simulink model "BLDCmotorControl_FOC_R2017b_fixdt"  (R2017b)
settings: Solver=FixedStepDiscrete  StartTime=0  StopTime=0.5  FixedStep=Ts  MaxStep=1e-6  RelTol=1e-6  AbsTol=1e-6  EnableMultiTasking=on
PreLoadFcn:
  | addpath(pwd);
  | addpath(genpath('01_Libraries'));
  | addpath(genpath('02_Figures'));
  | addpath(genpath('03_CreateParamTable'));
InitFcn:
  | init_model;
values from neighbouring files (symbols this model uses):
  a_elecAngle = 60    [init_model.m]
  a_elecPeriod = 360    [init_model.m]
  a_phaAdvMax = 25    [init_model.m]
  b_diagEna = 1    [init_model.m]
  b_fieldWeakEna = 0    [init_model.m]
  cf_currFilt = 0.12    [init_model.m]
  cf_idKi = 60 / (f_ctrl/3)    (= 0.01125)    [init_model.m]
  cf_idKp = 0.2    [init_model.m]
  cf_iqKi = 100 / (f_ctrl/3)    (= 0.01875)    [init_model.m]
  cf_iqKiLimProt = 60 / (f_ctrl/3)    (= 0.01125)    [init_model.m]
  cf_iqKp = 0.3    [init_model.m]
  cf_KbLimProt = 1000 / (f_ctrl/3)    (= 0.1875)    [init_model.m]
  cf_nKi = 20.4 / (f_ctrl/3)    (= 0.003825)    [init_model.m]
  cf_nKiLimProt = 20 / (f_ctrl/3)    (= 0.00375)    [init_model.m]
  cf_nKp = 1.18    [init_model.m]
  cf_speedCoef = round(f_ctrl * a_mechAngle * (pi/180) * (30/pi))    [init_model.m]
  CTRL_COM = 0    [init_model.m]
  CTRL_FOC = 2    [init_model.m]
  CTRL_SIN = 1    [init_model.m]
  dV_openRate = 1000 / (f_ctrl/3)    (= 0.1875)    [init_model.m]
  dz_cntTrnsDetHi = 40    [init_model.m]
  dz_cntTrnsDetLo = 20    [init_model.m]
  i_max = i_max * i_sca    (= 750)    [init_model.m]
  id_fieldWeakMax = 5 * i_sca    (= 250)    [init_model.m]
  iq_maxSca_M1 = sqrt(1 - iq_maxSca_XA.^2)    [init_model.m]
  n_commAcvLo = 15    [init_model.m]
  n_commDeacvHi = 30    [init_model.m]
  n_fieldWeakAuthHi = 400    [init_model.m]
  n_fieldWeakAuthLo = 300    [init_model.m]
  n_max = 1000    [init_model.m]
  n_polePairs = 15    [init_model.m]
  n_stdStillDet = 3    [init_model.m]
  OPEN_MODE = 0    [init_model.m]
  r_cos_M1 = cos((a_elecAngle_XA + 0)*(pi/180))    [init_model.m]
  r_errInpTgtThres = 600    [init_model.m]
  r_fieldWeakHi = 1500    [init_model.m]
  r_fieldWeakLo = 1000    [init_model.m]
  r_sin3PhaA_M1 = sin3Arm + A*r_sinPhaA_M1    [init_model.m]
  r_sin3PhaB_M1 = sin3Arm + A*r_sinPhaB_M1    [init_model.m]
  r_sin3PhaC_M1 = sin3Arm + A*r_sinPhaC_M1    [init_model.m]
  r_sin_M1 = sin((a_elecAngle_XA + 0)*(pi/180))    [init_model.m]
  SPD_MODE = 2    [init_model.m]
  t_errDequal = 1.80 * f_ctrl/3    (= 9600)    [init_model.m]
  t_errQual = 0.24 * f_ctrl/3    (= 1280)    [init_model.m]
  TRQ_MODE = 3    [init_model.m]
  Ts = 5e-6    (= 5e-06)    [init_model.m]
  Ts_ctrl = 6e-5    (= 6e-05)    [init_model.m]
  Vd_max = 1000 - V_margin    (= 900)    [init_model.m]
  vec_hallToPos = [0 2 0 1 4 3 5 0]    [init_model.m]
  VLT_MODE = 1    [init_model.m]
  Vq_max_M1 = sqrt(Vd_max^2 - Vq_max_XA.^2)    [init_model.m]
  z_commutMap_M1 = [-1 -1  0  1  1  0 ... (first row only)    [init_model.m]
  z_ctrlModReq = VLT_MODE    (= 1)    [init_model.m]
  z_ctrlTypSel = 2    [init_model.m]
  z_maxCntRst = 2000    [init_model.m]
  z_selPhaCurMeasABC = 0    [init_model.m]
undefined symbols (not defined in the file or in its folder): DiscIntNeverNeededParam, sigbuilder_block
libraries: BLDC_controller_Lib x15, simulink x14, powerlib x6, pePwmGenerator x1
(part 4 of 4)

== system BLDCmotorControl_FOC_R2017b_fixdt/BLDC_controller/F05_Field_Oriented_Control/Clarke_Transform/Clarke_PhasesBC ==
  note: Clarke Transform:
      | i_alpha = - i_phaB - i_phaC
      | i_beta = (1/sqrt(3)) * (i_phaB - i_phaC)
  i_phaB : Inport
  i_phaC : Inport  Port=2
  Action Port : ActionPort  ActionType=elseif
  Gain2 : Gain  Tag=struct('comment',struct('text','','placement',1),'logdata',struct('maxnumvals',inf,'plotchannels',[],'loggingmode',3,'channels',1),'output',struct('variable','','description','','name','$S_$B','width',1,'address','','max',NaN,'min',NaN,'class','default','type','CONTINUOUS','scaling','','lsb',1,'offset',0,'arb',0,'freeze',1,'unit','','autoscalingmode',1,'lowerheadroom',1,'upperheadroom',1,'headroomunit','bit','keepdatatype',1,'checkmin',0,'checkmax',0,'castoutput',0,'show',0),'gain',struct('variable','','description','','name','$S_$B_gain','width',1,'address','','max',NaN,'min',NaN,'class','default','type','CONTINUOUS','scaling','','lsb',1,'offset',0,'arb',0,'freeze',1,'unit','','keepdatatype',1,'value','1','scalar',0,'tolerance',1),'scalingvalid',0,'date',730486)  Gain=1/sqrt(3)  RndMeth=Zero  OutDataTypeStr=Inherit: Same as input
  Sum1 : Sum  Inputs=--  OutDataTypeStr=fixdt(1,16,4)  RndMeth=Simplest  SaturateOnIntegerOverflow=on
  Sum3 : Sum  Inputs=+-  OutDataTypeStr=fixdt(1,16,4)  RndMeth=Simplest  SaturateOnIntegerOverflow=on
  i_alphaBC : Outport
  i_betaBC : Outport  Port=2
  wires:
  [i_phaC] -> Sum1/2
  [i_phaB] -> Sum1/1
  [i_phaC] -> Sum3/2
  Gain2/1 -> i_betaBC/1
  Sum3/1 -> Gain2/1
  [i_phaB] -> Sum3/1
  Sum1/1 -> i_alphaBC/1
  i_phaB/1 -> [i_phaB]
  i_phaC/1 -> [i_phaC]

== system BLDCmotorControl_FOC_R2017b_fixdt/BLDC_controller/F05_Field_Oriented_Control/FOC/Open_Mode ==
  note: Just copy the target which will be reduced to 0 in the Input_Target_Sythesis function.
  r_inpTgtSca : Inport
  Action Port : ActionPort  ActionType=default
  Vq_Open : Outport
  wires:
  r_inpTgtSca/1 -> Vq_Open/1

== system BLDCmotorControl_FOC_R2017b_fixdt/BLDC_controller/F05_Field_Oriented_Control/FOC/Speed_Mode ==
  note: The input is scaled, so already between [n_min, n_max]
  r_inpTgtSca : Inport
  Vq_max : Inport  Port=2
  Vq_min : Inport  Port=3
  n_mot : Inport  Port=4
  iq_limProtErr : Inport  Port=5
  Action Port : ActionPort  ActionType=case
  PI_clamp_fixdt : BLDC_controller_Lib/PI_clamp_fixdt  SystemSampleTime=-1
  Sum3 : Sum  Inputs=|+-  RndMeth=Simplest  SaturateOnIntegerOverflow=on
  cf_nKi : Constant  Value=cf_nKi  VectorParams1D=off  OutDataTypeStr=fixdt(0,16,16)
  cf_nKp : Constant  Value=cf_nKp  OutDataTypeStr=fixdt(0,16,12)
  Vq_Spd : Outport
  wires:
  cf_nKi/1 -> PI_clamp_fixdt/3
  cf_nKp/1 -> PI_clamp_fixdt/2
  [n_mot] -> Sum3/2
  Sum3/1 -> PI_clamp_fixdt/1
  r_inpTgtSca/1 -> [r_inpTgtSca]
  Vq_max/1 -> [Vq_max]
  Vq_min/1 -> [Vq_min]
  n_mot/1 -> [n_mot]
  [r_inpTgtSca] -> Sum3/1
  iq_limProtErr/1 -> [iq_limProtErr]
  [iq_limProtErr] -> PI_clamp_fixdt/6
  PI_clamp_fixdt/1 -> Vq_Spd/1
  [Vq_min] -> PI_clamp_fixdt/5
  [Vq_max] -> PI_clamp_fixdt/4

== system BLDCmotorControl_FOC_R2017b_fixdt/BLDC_controller/F05_Field_Oriented_Control/FOC/Torque_Mode ==
  r_inpTgtSca : Inport
  Vq_max : Inport  Port=2
  Vq_min : Inport  Port=3
  iq : Inport  Port=4
  iq_max : Inport  Port=5
  iq_min : Inport  Port=6
  Vq_nLimProtMax : Inport  Port=7
  Action Port : ActionPort  ActionType=case
  Gain4 : Gain  Tag=struct('comment',struct('text','','placement',1),'logdata',struct('maxnumvals',inf,'plotchannels',[],'loggingmode',3,'channels',1),'output',struct('variable','','description','','name','$S_$B','width',1,'address','','max',NaN,'min',NaN,'class','default','type','CONTINUOUS','scaling','','lsb',1,'offset',0,'arb',0,'freeze',1,'unit','','autoscalingmode',1,'lowerheadroom',1,'upperheadroom',1,'headroomunit','bit','keepdatatype',1,'checkmin',0,'checkmax',0,'castoutput',0,'show',0),'gain',struct('variable','','description','','name','$S_$B_gain','width',1,'address','','max',NaN,'min',NaN,'class','default','type','CONTINUOUS','scaling','','lsb',1,'offset',0,'arb',0,'freeze',1,'unit','','keepdatatype',1,'value','1','scalar',0,'tolerance',1),'scalingvalid',0,'date',730486)  Gain=-1  RndMeth=Zero  OutDataTypeStr=Inherit: Same as input  ParamDataTypeStr=Inherit: Same as input
  MinMax1 : MinMax  Inputs=2
  MinMax2 : MinMax  Function=max  Inputs=2
  PI_clamp_fixdt : BLDC_controller_Lib/PI_clamp_fixdt  SystemSampleTime=-1
  Saturation Dynamic1 : simulink/Discontinuities/Saturation Dynamic  OutMin=[]  OutMax=[]  OutDataTypeStr=Inherit: Same as second input  OutDataType=fixdt(1, 16)  OutScaling=2^-10  DoSatur=off
  Sum2 : Sum  Inputs=|+-  RndMeth=Simplest  SaturateOnIntegerOverflow=on
  cf_iqKi : Constant  Value=cf_iqKi  OutDataTypeStr=fixdt(0,16,16)
  cf_iqKp : Constant  Value=cf_iqKp  OutDataTypeStr=fixdt(0,16,12)
  constant2 : Constant  Value=0  OutDataTypeStr=Inherit: Inherit via back propagation
  Vq_Trq : Outport
  wires:
  Vq_max/1 -> [Vq_max]
  r_inpTgtSca/1 -> [r_inpTgtSca]
  Vq_min/1 -> [Vq_min]
  iq/1 -> [iq]
  iq_min/1 -> [iq_min]
  iq_max/1 -> [iq_max]
  Vq_nLimProtMax/1 -> [Vq_nLimProtMax]
  [r_inpTgtSca] -> Saturation Dynamic1/2
  constant2/1 -> PI_clamp_fixdt/6
  Saturation Dynamic1/1 -> Sum2/1
  PI_clamp_fixdt/1 -> Vq_Trq/1
  [iq_max] -> Saturation Dynamic1/1
  [iq_min] -> Saturation Dynamic1/3
  cf_iqKp/1 -> PI_clamp_fixdt/2
  Sum2/1 -> PI_clamp_fixdt/1
  [iq] -> Sum2/2
  [Vq_minTrq] -> PI_clamp_fixdt/5
  [Vq_maxTrq] -> PI_clamp_fixdt/4
  cf_iqKi/1 -> PI_clamp_fixdt/3
  [Vq_nLimProtMax] -> MinMax1/2, Gain4/1
  [Vq_max] -> MinMax1/1
  Gain4/1 -> MinMax2/1
  [Vq_min] -> MinMax2/2
  MinMax1/1 -> [Vq_maxTrq]
  MinMax2/1 -> [Vq_minTrq]

== system BLDCmotorControl_FOC_R2017b_fixdt/BLDC_controller/F05_Field_Oriented_Control/FOC/Vd_Calculation ==
  id_Tgt : Inport
  id : Inport  Port=2
  Vd_max : Inport  Port=3
  Vd_min : Inport  Port=4
  id_max : Inport  Port=5
  id_min : Inport  Port=6
  Action Port : ActionPort  ActionType=then
  PI_clamp_fixdt : BLDC_controller_Lib/PI_clamp_fixdt  SystemSampleTime=-1
  Saturation Dynamic : simulink/Discontinuities/Saturation Dynamic  OutMin=[]  OutMax=[]  OutDataTypeStr=Inherit: Same as second input  OutDataType=fixdt(1, 16)  OutScaling=2^-10  DoSatur=off
  Sum3 : Sum  Inputs=|+-  RndMeth=Simplest  SaturateOnIntegerOverflow=on
  cf_idKi1 : Constant  Value=cf_idKi  OutDataTypeStr=fixdt(0,16,16)
  cf_idKp1 : Constant  Value=cf_idKp  OutDataTypeStr=fixdt(0,16,12)
  constant1 : Constant  Value=0  OutDataTypeStr=Inherit: Inherit via back propagation
  Vd : Outport
  wires:
  [id] -> Sum3/2
  [id_Tgt] -> Saturation Dynamic/2
  id_Tgt/1 -> [id_Tgt]
  id/1 -> [id]
  Vd_min/1 -> [Vd_min]
  Vd_max/1 -> [Vd_max]
  id_max/1 -> [id_max]
  id_min/1 -> [id_min]
  Saturation Dynamic/1 -> Sum3/1
  [id_max] -> Saturation Dynamic/1
  [id_min] -> Saturation Dynamic/3
  Sum3/1 -> PI_clamp_fixdt/1
  PI_clamp_fixdt/1 -> Vd/1
  cf_idKp1/1 -> PI_clamp_fixdt/2
  cf_idKi1/1 -> PI_clamp_fixdt/3
  constant1/1 -> PI_clamp_fixdt/6
  [Vd_min] -> PI_clamp_fixdt/5
  [Vd_max] -> PI_clamp_fixdt/4

== system BLDCmotorControl_FOC_R2017b_fixdt/BLDC_controller/F05_Field_Oriented_Control/FOC/Voltage_Mode ==
  r_inpTgtSca : Inport
  r_inpTgtScaAbs : Inport  Port=2
  Vq_max : Inport  Port=3
  Vq_min : Inport  Port=4
  r_iqLimProtMax : Inport  Port=5
  r_nLimProtMax : Inport  Port=6
  Action Port : ActionPort  ActionType=case
  Divide1 : Product  Inputs=**  RndMeth=Simplest  OutDataTypeStr=Inherit: Same as first input
  MinMax : MinMax  Inputs=3
  Saturation Dynamic1 : simulink/Discontinuities/Saturation Dynamic  OutMin=[]  OutMax=[]  OutDataTypeStr=Inherit: Same as second input  OutDataType=fixdt(1, 16)  OutScaling=2^-10  DoSatur=off
  SignDeltaU2 : Signum  DisableCoverage=on
  Signal Conversion2 : SignalConversion  OverrideOpt=off
  Vq_Vlt : Outport
  wires:
  r_inpTgtSca/1 -> [r_inpTgtSca]
  [Vq_min] -> Saturation Dynamic1/3
  [Vq_max] -> Saturation Dynamic1/1
  Vq_max/1 -> [Vq_max]
  Vq_min/1 -> [Vq_min]
  r_iqLimProtMax/1 -> [r_iqLimProtMax]
  r_nLimProtMax/1 -> [r_nLimProtMax]
  Signal Conversion2/1 -> Vq_Vlt/1
  Saturation Dynamic1/1 -> Signal Conversion2/1
  [r_nLimProtMax] -> MinMax/3
  [r_iqLimProtMax] -> MinMax/2
  r_inpTgtScaAbs/1 -> [r_inpTgtScaAbs]
  [r_inpTgtScaAbs] -> MinMax/1
  [r_inpTgtSca] -> SignDeltaU2/1
  MinMax/1 -> Divide1/1
  SignDeltaU2/1 -> Divide1/2
  Divide1/1 -> Saturation Dynamic1/2

== system BLDCmotorControl_FOC_R2017b_fixdt/BLDC_controller/F05_Field_Oriented_Control/Motor_Limitations/Speed_Mode_Protection ==
  iq : Inport
  iq_max : Inport  Port=2
  iq_min : Inport  Port=3
  Action Port : ActionPort  ActionType=case
  Divide1 : Product  Inputs=**  OutDataTypeStr=fixdt(1,32,20)  RndMeth=Simplest
  Saturation Dynamic : simulink/Discontinuities/Saturation Dynamic  OutMin=[]  OutMax=[]  OutDataTypeStr=Inherit: Same as second input  OutDataType=fixdt(1, 16)  OutScaling=2^-10  DoSatur=off
  Sum3 : Sum  Inputs=|+-  RndMeth=Simplest
  cf_iqKiLimProt : Constant  Value=cf_iqKiLimProt  OutDataTypeStr=fixdt(0,16,16)
  iq_limProtErr : Outport  InitialOutput=0
  wires:
  iq/1 -> Sum3/2, Saturation Dynamic/2
  Saturation Dynamic/1 -> Sum3/1
  iq_max/1 -> Saturation Dynamic/1
  iq_min/1 -> Saturation Dynamic/3
  cf_iqKiLimProt/1 -> Divide1/2
  Divide1/1 -> iq_limProtErr/1
  Sum3/1 -> Divide1/1

== system BLDCmotorControl_FOC_R2017b_fixdt/BLDC_controller/F05_Field_Oriented_Control/Motor_Limitations/Torque_Mode_Protection ==
  n_motAbs : Inport
  n_max : Inport  Port=2
  Vq_max : Inport  Port=3
  Action Port : ActionPort  ActionType=case
  Constant1 : Constant  Value=0  OutDataTypeStr=Inherit: Inherit via back propagation
  I_backCalc_fixdt : BLDC_controller_Lib/I_backCalc_fixdt  yInit=0
      settings: AttributesFormatString=Ini=%<yInit>
  Sum1 : Sum  Inputs=+-  RndMeth=Simplest  OutDataTypeStr=Inherit: Same as first input
  cf_KbLimProt : Constant  Value=cf_KbLimProt  OutDataTypeStr=fixdt(0,16,12)
  cf_nKiLimProt : Constant  Value=cf_nKiLimProt  OutDataTypeStr=fixdt(0,16,16)
  Vq_nLimProtMax : Outport  InitialOutput=0
  wires:
  n_motAbs/1 -> [n_motAbs]
  n_max/1 -> [n_max]
  Sum1/1 -> I_backCalc_fixdt/1
  [n_motAbs] -> Sum1/2
  Constant1/1 -> I_backCalc_fixdt/5
  [n_max] -> Sum1/1
  cf_nKiLimProt/1 -> I_backCalc_fixdt/2
  cf_KbLimProt/1 -> I_backCalc_fixdt/3
  [Vq_max] -> I_backCalc_fixdt/4
  I_backCalc_fixdt/1 -> Vq_nLimProtMax/1
  Vq_max/1 -> [Vq_max]

== system BLDCmotorControl_FOC_R2017b_fixdt/BLDC_controller/F05_Field_Oriented_Control/Motor_Limitations/Voltage_Mode_Protection ==
  r_inpTgtScaAbs : Inport
  iqAbs : Inport  Port=2
  iq_max : Inport  Port=3
  n_motAbs : Inport  Port=4
  n_max : Inport  Port=5
  Action Port : ActionPort  ActionType=case
  Constant : Constant  Value=0  OutDataTypeStr=Inherit: Inherit via back propagation
  Constant1 : Constant  Value=0  OutDataTypeStr=Inherit: Inherit via back propagation
  I_backCalc_fixdt : BLDC_controller_Lib/I_backCalc_fixdt  yInit=0
      settings: AttributesFormatString=Ini=%<yInit>
  I_backCalc_fixdt1 : BLDC_controller_Lib/I_backCalc_fixdt  yInit=0
      settings: AttributesFormatString=Ini=%<yInit>
  Sum1 : Sum  Inputs=+-  RndMeth=Simplest  OutDataTypeStr=Inherit: Same as first input
  Sum2 : Sum  Inputs=+-  RndMeth=Simplest  OutDataTypeStr=Inherit: Same as first input
  cf_KbLimProt : Constant  Value=cf_KbLimProt  OutDataTypeStr=fixdt(0,16,12)
  cf_iqKiLimProt : Constant  Value=cf_iqKiLimProt  OutDataTypeStr=fixdt(0,16,16)
  cf_nKiLimProt : Constant  Value=cf_nKiLimProt  OutDataTypeStr=fixdt(0,16,16)
  r_iqLimProtMax : Outport  InitialOutput=0
  r_nLimProtMax : Outport  Port=2  InitialOutput=0
  wires:
  iq_max/1 -> [iq_max]
  iqAbs/1 -> [iqAbs]
  n_max/1 -> [n_max]
  n_motAbs/1 -> [n_motAbs]
  Sum2/1 -> I_backCalc_fixdt/1
  [iq_max] -> Sum2/1
  [iqAbs] -> Sum2/2
  Constant/1 -> I_backCalc_fixdt/5
  [r_inpTgtScaAbs] -> I_backCalc_fixdt1/4, I_backCalc_fixdt/4
  cf_iqKiLimProt/1 -> I_backCalc_fixdt/2
  cf_KbLimProt/1 -> I_backCalc_fixdt1/3, I_backCalc_fixdt/3
  [r_iqLimProtMax] -> r_iqLimProtMax/1
  I_backCalc_fixdt/1 -> [r_iqLimProtMax]
  [r_nLimProtMax] -> r_nLimProtMax/1
  I_backCalc_fixdt1/1 -> [r_nLimProtMax]
  cf_nKiLimProt/1 -> I_backCalc_fixdt1/2
  Constant1/1 -> I_backCalc_fixdt1/5
  [n_motAbs] -> Sum1/2
  [n_max] -> Sum1/1
  Sum1/1 -> I_backCalc_fixdt1/1
  r_inpTgtScaAbs/1 -> [r_inpTgtScaAbs]

== system BLDCmotorControl_FOC_R2017b_fixdt/BLDC_controller/F06_Control_Type_Management/SIN_Method/Final_Phase_Advance_Calculation ==
  note: Phase Advance / Field Weakening
  a_elecAngle : Inport
  z_dir : Inport  Port=2
  r_fieldWeak : Inport  Port=3
  Modulo_fixdt : BLDC_controller_Lib/Modulo_fixdt
  Mux : Mux  Inputs=2
  Product2 : Product  RndMeth=Simplest  OutDataTypeStr=Inherit: Same as first input
  Scope : Scope  NumInputPorts=2
  Sum3 : Sum  RndMeth=Simplest  OutDataTypeStr=Inherit: Same as first input
  Switch_PhaAdv : Switch  Criteria=u2 ~= 0  OutDataTypeStr=Inherit: Inherit via back propagation  RndMeth=Zero
  a_elecPeriod2 : Constant  Value=a_elecPeriod  OutDataTypeStr=Inherit: Inherit via back propagation
  b_fieldWeakEna : Constant  Value=b_fieldWeakEna  OutDataTypeStr=boolean
  a_elecAngleAdv : Outport  OutputWhenDisabled=reset  InitialOutput=0
  wires:
  [r_fieldWeak] -> Product2/1
  [z_dir] -> Product2/2
  z_dir/1 -> [z_dir]
  Mux/1 -> Scope/1
  Modulo_fixdt/1 -> Switch_PhaAdv/1
  [a_elecAngleAdv] -> a_elecAngleAdv/1
  [r_fieldWeak] -> Scope/2
  [a_elecAngle] -> Sum3/1
  a_elecPeriod2/1 -> Modulo_fixdt/2
  Sum3/1 -> Modulo_fixdt/1
  r_fieldWeak/1 -> [r_fieldWeak]
  a_elecAngle/1 -> [a_elecAngle]
  b_fieldWeakEna/1 -> Switch_PhaAdv/2
  Product2/1 -> Sum3/2
  [a_elecAngle] -> Mux/1
  [a_elecAngle] -> Switch_PhaAdv/3
  Switch_PhaAdv/1 -> [a_elecAngleAdv]
  [a_elecAngleAdv] -> Mux/2

== stateflow chart BLDCmotorControl_FOC_R2017b_fixdt/BLDC_controller/F03_Control_Mode_Manager/F03_02_Control_Mode_Manager ==
  state OPEN
    entry:
    z_ctrlMod = OPEN_MODE;
  state ACTIVE
    state TORQUE_MODE
      entry:
      z_ctrlMod = TRQ_MODE;
    state SPEED_MODE
      entry:
      z_ctrlMod = SPD_MODE;
    state VOLTAGE_MODE
      entry:
      z_ctrlMod = VLT_MODE;
    (default) -> (junction 7)
    TORQUE_MODE -> ACTIVE : [~b_toTrqMod]
    (junction 7) -> TORQUE_MODE [order 1] : [b_toTrqMod]
    (junction 7) -> (junction 8) [order 2]
    SPEED_MODE -> ACTIVE : [~b_toSpdMod]
    (junction 8) -> SPEED_MODE [order 1] : [b_toSpdMod]
    (junction 8) -> (junction 29) [order 2]
    VOLTAGE_MODE -> ACTIVE : [b_toTrqMod || ...
        | b_toSpdMod]
    (junction 29) -> VOLTAGE_MODE
  (default) -> OPEN
  OPEN -> ACTIVE : [b_toActive]
  ACTIVE -> OPEN : [b_toOpen]
  data: b_toOpen input boolean; b_toActive input boolean; b_toSpdMod input boolean; z_ctrlMod output uint8; OPEN_MODE constant uint8 =OPEN_MODE; TRQ_MODE constant uint8 =TRQ_MODE; SPD_MODE constant uint8 =SPD_MODE; VLT_MODE constant uint8 =VLT_MODE; b_toTrqMod input boolean
